simulink model "QuarterCarSuspensionModel"  (R2025b)
settings: Solver=ode23t  StartTime=0.0  StopTime=20  RelTol=1e-3
values from neighbouring files (symbols this model uses):
  c = 100    [initialize_LF.m]    (also in initialize_PID.m = 300)
  k = 10000    [initialize_LF.m]    (also in initialize_PID.m)
  m = 200    [initialize_LF.m]    (also in initialize_PID.m = 300)
settings Model: Creator=kanch  LastModifiedBy=kanch

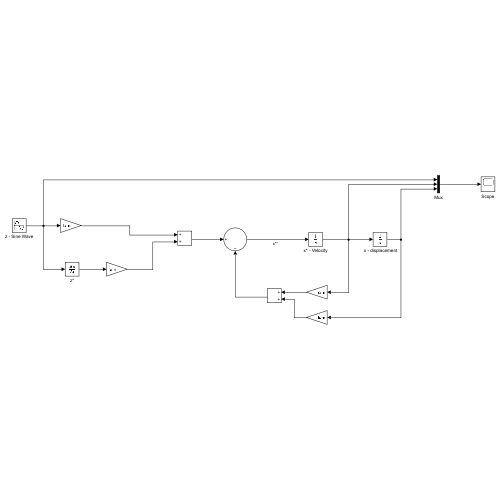
[thumbnail: Simulink's stored preview of the top-level diagram]
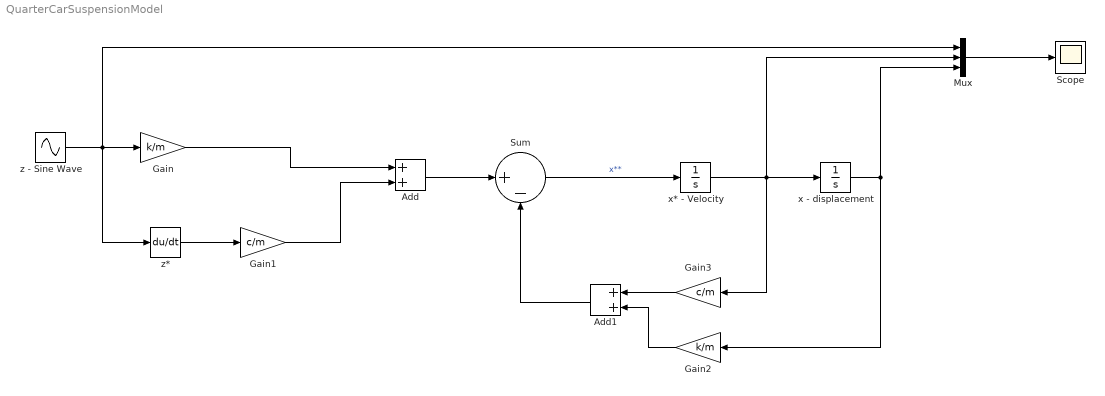
== system QuarterCarSuspensionModel ==
  " x - displacement" : Integrator
  Add : Sum
  Add1 : Sum
  Gain : Gain  Gain=k/m
  Gain1 : Gain  Gain=c/m
  Gain2 : Gain  Gain=k/m
  Gain3 : Gain  Gain=c/m
  Mux : Mux  Inputs=3
  Scope : Scope
      settings: ActiveDisplayYMinimum=-2.1500339777227713  ActiveDisplayYMaximum=2.5922864931021494
  Sum : Sum  Inputs=|+-
  x* - Velocity : Integrator
  z - Sine Wave : Sin  SampleTime=0
  z* : Derivative
  wires:
  z - Sine Wave/1 -> Mux/1, z*/1, Gain/1
  z*/1 -> Gain1/1
  Gain/1 -> Add/1
  Gain1/1 -> Add/2
  Add/1 -> Sum/1
  Sum/1 -> x* - Velocity/1  "x**"
  x* - Velocity/1 -> Mux/2, Gain3/1, " x - displacement"/1
  Add1/1 -> Sum/2
  Gain3/1 -> Add1/1
  Gain2/1 -> Add1/2
  " x - displacement"/1 -> Gain2/1, Mux/3
  Mux/1 -> Scope/1
